simulink model "model1LAB1"  (R2020a)
settings: Solver=VariableStepAuto  StartTime=0.0  StopTime=10.0  RelTol=1e-3
libraries: commrandsrc3 x1
settings Model: Creator=Sameer  LastModifiedBy=Sameer

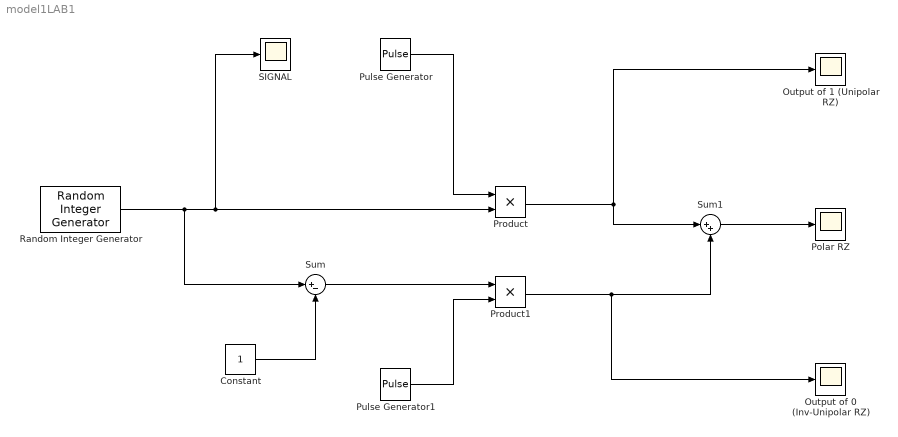
== system model1LAB1 ==
  Constant : Constant
  Output of 0 (Inv-Unipolar RZ) : Scope
  Output of 1 (Unipolar RZ) : Scope
  Polar RZ : Scope
  Product : Product
  Product1 : Product
  Pulse Generator : DiscretePulseGenerator  PulseType=Time based  Period=10  PulseWidth=5
  Pulse Generator1 : DiscretePulseGenerator  PulseType=Time based  Period=10  PulseWidth=5
  Random Integer Generator : commrandsrc3/Random Integer Generator  SetSize=8  SeedSource=Auto  Seed=0  SampleTime=1  SamplesPerFrame=1  OutputDataType=double  SimulateUsing=Interpreted execution
  SIGNAL : Scope
      settings: Description=SIGNAL
  Sum : Sum  Inputs=|+-
  Sum1 : Sum  Inputs=|++
  wires:
  Constant/1 -> Sum/2
  Random Integer Generator/1 -> Sum/1, SIGNAL/1, Product/2
  Pulse Generator/1 -> Product/1
  Sum/1 -> Product1/1
  Pulse Generator1/1 -> Product1/2
  Product1/1 -> Output of 0 (Inv-Unipolar RZ)/1, Sum1/2
  Product/1 -> Sum1/1, Output of 1 (Unipolar RZ)/1
  Sum1/1 -> Polar RZ/1
